simulink model "mPowerLossDistributorPassiveCooling"  (R2021b)
settings: Solver=VariableStepAuto  StartTime=0.0  StopTime=10.0  RelTol=1e-3
model workspace (MAT data in the model file):
  AdjacencyMat = [0 0 0 0 0 0 0 0 0 0 0 0 ... (15129 elements, 123x123)]
  CapMat = [1e+20 2196.70091586 387.653102799 193.8265514 1962.34710525 387.653102799 193.8265514 1962.34710525 1266.59353814 268.053957132 416.539515956 175.715078 ... (123 elements, 123x1)]
  CoolantArrayIdxs = [20 21 22 23 24 25 26 27 35 36 37 84 ... (19 elements, 19x1)]
  Friction_Loss_Mat = [0 0 0 0 0 0 0 0 0 0 0 0 ... (2340 elements, 39x60)]
  InletCoolIdxs = [37; 38]
  Iron_Loss_Rotor_Back_Iron_Mat = [0.0117485795538 0.0197051847397 0.0244700561647 0.0255532537599 0.0239976928195 0.0207690118754 0.0168550814705 0.0133554634632 0.01151831468 0.0120080610473 0.0141635691716 0.0169722368466 ... (2340 elements, 39x60)]
  Iron_Loss_Rotor_Pole_Mat = [1.4581490918 1.4537473697 1.43037570585 1.39187577753 1.34319900564 1.28804676124 1.2293784806 1.16971068454 1.11123984852 1.0549546703 0.999931477749 0.94446781724 ... (2340 elements, 39x60)]
  Iron_Loss_Rotor_Tooth_Mat = [0 0 0 0 0 0 0 0 0 0 0 0 ... (2340 elements, 39x60)]
  Iron_Loss_Stator_Back_Iron_Mat = [38.4149877088 37.6503107125 36.6652845221 35.5768425978 34.4225640875 33.2346156756 32.0443324124 30.8866766706 29.801209009 28.7963723188 27.8072961338 26.7363012626 ... (2340 elements, 39x60)]
  Iron_Loss_Stator_Tooth_Mat = [42.0487318978 41.0399202886 40.1567907901 39.4070106899 38.6872815615 37.9480215396 37.175663609 36.3826322946 35.5969122241 34.8195499408 33.9921719085 33.0420249153 ... (2340 elements, 39x60)]
  LossDistrForEachType = [0 0 0 0 0 0 0 0 0 0 0 0 ... (1968 elements, 16x123)]
  Magnet_Loss_Mat = [0.0992355707119 0.0926361497593 0.0866339598393 0.0816717050449 0.0772717421391 0.0730472022398 0.0686189288913 0.0635413555728 0.0572450430654 0.0495346500988 0.0410747136719 0.0327097040848 ... (2340 elements, 39x60)]
  OutletCoolIdxs = [20; 107]
  Rotor_Cage_Loss_Mat = [0 0 0 0 0 0 0 0 0 0 0 0 ... (2340 elements, 39x60)]
  ShaftTorqueVec = [-285.363175319 -270.469371582 -255.575567846 -240.681764109 -225.787960373 -210.894156636 -196.0003529 -181.106549163 -166.212745427 -151.31894169 -136.425137954 -121.531334217 ... (39 elements, 1x39)]
  SpeedVec = [500 661.016949153 822.033898305 983.050847458 1144.06779661 1305.08474576 1466.10169492 1627.11864407 1788.13559322 1949.15254237 2110.16949153 2271.18644068 ... (60 elements, 1x60)]
  StateSpaceND : object (value not decoded)
  StatorCopperTempCoefResistivity = 0.00393
  Stator_Copper_Loss_Mat = [4036.39837515 3610.67609702 3178.68722837 2791.06956208 2441.07338047 2123.72912642 1835.28722535 1572.85477291 1334.16141597 1117.77314243 921.650266023 744.483696972 ... (2340 elements, 39x60)]
  Stray_Load_Loss_Mat = [0 0 0 0 0 0 0 0 0 0 0 0 ... (2340 elements, 39x60)]
  Stray_Loss_Stator_Iron_Proportion = 0.95
  Tgiven = 20
  TnodesInit = [25 25 25 25 25 25 25 25 25 25 25 25 ... (123 elements, 123x1)]
  Tsim = 20
  Windage_Loss_Mat = [0 0 0 0 0 0 0 0 0 0 0 0 ... (2340 elements, 39x60)]
  armatureCopperLossVal = 35
  backIronLossVal = 15
  magnetLossVal = 12
  speedVal = 2000
  toothIronLossVal = 25
  torqueVal = 20
libraries: mcadROM_lib x2
(part 2 of 2)

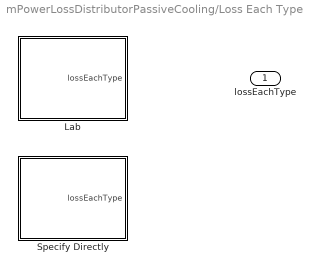
== system mPowerLossDistributorPassiveCooling/Loss Each Type ==
  Lab : Subsystem  VariantControl=Lab
  Specify Directly : Subsystem  VariantControl=Specify Directly
  lossEachType : Outport

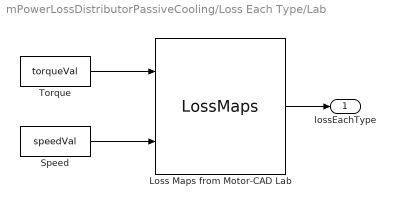
== system mPowerLossDistributorPassiveCooling/Loss Each Type/Lab ==
  Loss Maps from Motor-CAD Lab : mcadROM_lib/LossMaps  ShaftTorqueVec=ShaftTorqueVec  SpeedVec=SpeedVec  Stator_Copper_Loss_Mat=Stator_Copper_Loss_Mat  Rotor_Cage_Loss_Mat=Rotor_Cage_Loss_Mat  Iron_Loss_Stator_Back_Iron_Mat=Iron_Loss_Stator_Back_Iron_Mat  Iron_Loss_Stator_Tooth_Mat=Iron_Loss_Stator_Tooth_Mat  Stray_Loss_Stator_Iron_Proportion=Stray_Loss_Stator_Iron_Proportion  Stray_Load_Loss_Mat=Stray_Load_Loss_Mat  Magnet_Loss_Mat=Magnet_Loss_Mat  Iron_Loss_Rotor_Pole_Mat=Iron_Loss_Rotor_Pole_Mat  Iron_Loss_Rotor_Back_Iron_Mat=Iron_Loss_Rotor_Back_Iron_Mat  Iron_Loss_Rotor_Tooth_Mat=Iron_Loss_Rotor_Tooth_Mat  Friction_Loss_Mat=Friction_Loss_Mat  Windage_Loss_Mat=Windage_Loss_Mat
  Speed : Constant  Value=speedVal
  Torque : Constant  Value=torqueVal
  lossEachType : Outport
  wires:
  Torque/1 -> Loss Maps from Motor-CAD Lab/1
  Speed/1 -> Loss Maps from Motor-CAD Lab/2
  Loss Maps from Motor-CAD Lab/1 -> lossEachType/1

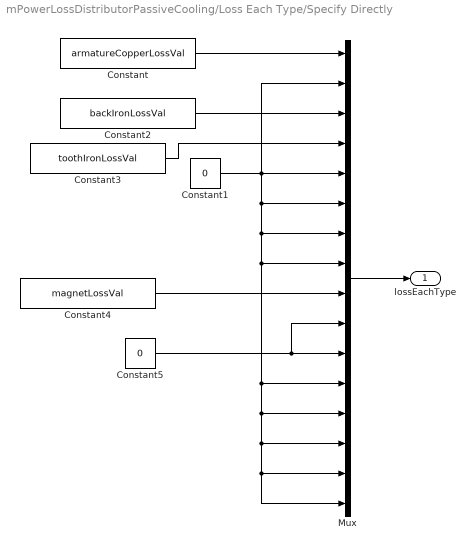
== system mPowerLossDistributorPassiveCooling/Loss Each Type/Specify Directly ==
  Constant : Constant  Value=armatureCopperLossVal
  Constant1 : Constant  Value=0
  Constant2 : Constant  Value=backIronLossVal
  Constant3 : Constant  Value=toothIronLossVal
  Constant4 : Constant  Value=magnetLossVal
  Constant5 : Constant  Value=0
  Mux : Mux  Inputs=16
  lossEachType : Outport
  wires:
  Mux/1 -> lossEachType/1
  Constant/1 -> Mux/1
  Constant1/1 -> Mux/16, Mux/15, Mux/14, Mux/13, Mux/12, Mux/8, Mux/7, Mux/6, Mux/2, Mux/5
  Constant2/1 -> Mux/3
  Constant3/1 -> Mux/4
  Constant4/1 -> Mux/9
  Constant5/1 -> Mux/10, Mux/11
